simulink model "fixed_4"  (Simulink 4.00)
settings: Solver=ode45  SolverMode=SingleTasking  StartTime=0.0  StopTime=10.0  RelTol=1e-3  AbsTol=1e-6
settings Model: LastModifiedBy=Administrator  OutputOption=SpecifiedOutputTimes  OutputTimes=[0:0.01:10]  BlockReductionOpt=off

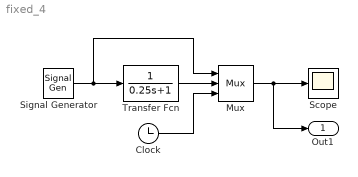
== system fixed_4 ==
  Clock : Clock
      settings: DisplayTime=off  Decimation=10
  Mux : Mux  Inputs=3
      settings: DisplayOption=none
  Scope : Scope
      settings: TickLabels=on  TimeRange=auto  YMin=-5  YMax=5  SaveToWorkspace=off  SaveName=ScopeData  DataFormat=Array  LimitDataPoints=on  MaxDataPoints=5000
  Signal Generator : SignalGenerator  WaveForm=square  Amplitude=1  Frequency=0.5  Units=Hertz
  Transfer Fcn : TransferFcn  Numerator=[1]  Denominator=[0.25 1]  Realization=auto  AbsoluteTolerance=auto
  Out1 : Outport  Port=1
  wires:
  Transfer Fcn/1 -> Mux/2
  Signal Generator/1 -> Transfer Fcn/1, Mux/1
  Mux/1 -> Out1/1, Scope/1
  Clock/1 -> Mux/3
